simulink model "ss_canonical_diagram"  (R2025b)
settings: Solver=FixedStepDiscrete  StartTime=0.0  StopTime=50  FixedStep=1  RelTol=1e-3
settings Model: Creator=avent  LastModifiedBy=avent

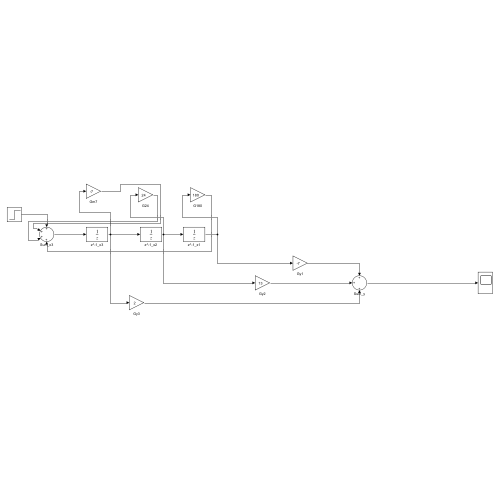
[thumbnail: Simulink's stored preview of the top-level diagram]
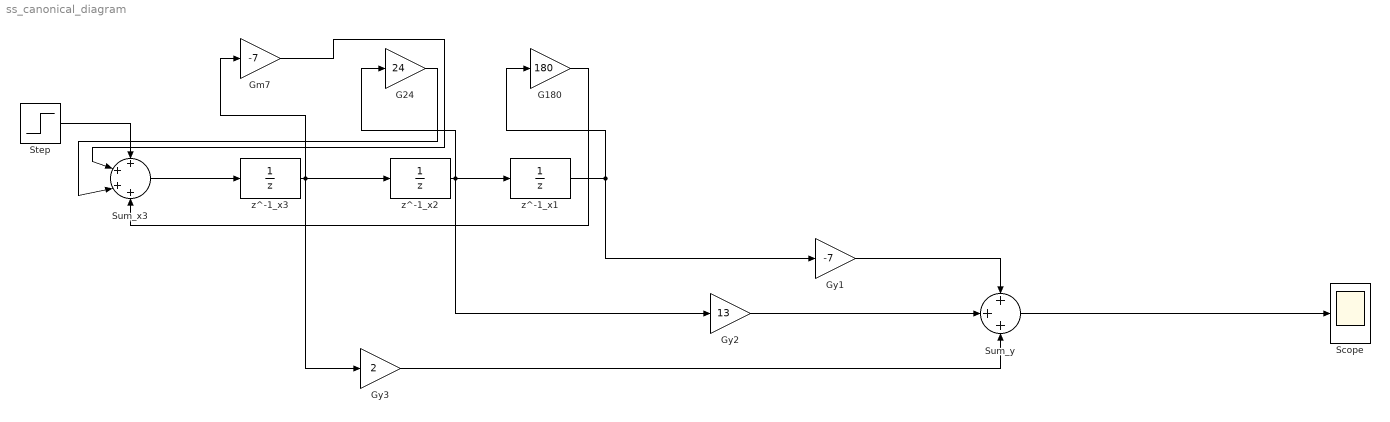
== system ss_canonical_diagram ==
  G180 : Gain  Gain=180
  G24 : Gain  Gain=24
  Gm7 : Gain  Gain=-7
  Gy1 : Gain  Gain=-7
  Gy2 : Gain  Gain=13
  Gy3 : Gain  Gain=2
  Scope : Scope
  Step : Step  Time=0  SampleTime=1
  Sum_x3 : Sum  Inputs=++++
  Sum_y : Sum  Inputs=+++
  z^-1_x1 : UnitDelay  HasFrameUpgradeWarning=on
  z^-1_x2 : UnitDelay  HasFrameUpgradeWarning=on
  z^-1_x3 : UnitDelay  HasFrameUpgradeWarning=on
  wires:
  Step/1 -> Sum_x3/1
  Sum_x3/1 -> z^-1_x3/1
  z^-1_x3/1 -> z^-1_x2/1, Gm7/1, Gy3/1
  z^-1_x2/1 -> z^-1_x1/1, G24/1, Gy2/1
  z^-1_x1/1 -> G180/1, Gy1/1
  Gm7/1 -> Sum_x3/2
  G24/1 -> Sum_x3/3
  G180/1 -> Sum_x3/4
  Gy1/1 -> Sum_y/1
  Gy2/1 -> Sum_y/2
  Gy3/1 -> Sum_y/3
  Sum_y/1 -> Scope/1
